simulink model "MonarcoHATdemo_exec"  (Simulink 3.00)
libraries: execlib x6

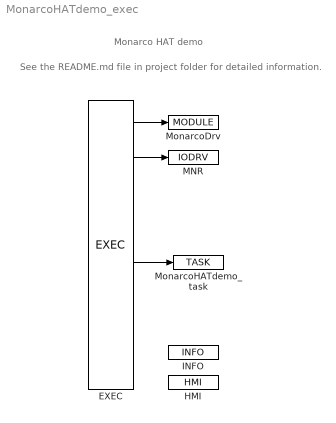
== system MonarcoHATdemo_exec ==
  note: See the README.md file in project
      | folder for detailed information.
  note: Monarco HAT demo
  EXEC : execlib/EXEC  target=Generic target device  tick=0.01  ntick0=1  ntick1=50  ntick2=100  ntick3=1200  pri0=5  pri1=9  pri2=13  pri3=18
  HMI : execlib/HMI  IncludeHMI=on  HmiDir=hmi  SourceDir=hmisrc  GenerateWebWatch=off  GenerateRexHMI=on  RedirectToHMI=on  Compression=off
  INFO : execlib/INFO  Title=Monarco HAT demo example  Author=REX Controls s.r.o.  Description=Monarco HAT demo example
  MNR : execlib/IODRV  module=MonarcoDrv  classname=MonarcoHatDrv  cfgname=monarcohat.rio  factor=1  stack=10240  pri=3  timer=off
  MonarcoDrv : execlib/MODULE
  MonarcoHATdemo_task : execlib/TASK  factor=1  start=0  stop=1  stack=10240  MDLOPEN=on
  wires:
  EXEC/1 -> MonarcoDrv/1
  EXEC/2 -> MNR/1
  EXEC/5 -> MonarcoHATdemo_task/1
